simulink model "Component_1"  (R2024a)
settings: Solver=VariableStepAuto  StartTime=0.0  StopTime=10.0  RelTol=1e-3
undefined symbols (not defined in the file or in its folder): canChannel
libraries: canmsglib x4, canlib x2
settings Model: DataDictionary=BMS_System_dict1.sldd  Creator=hirah  LastModifiedBy=hirah

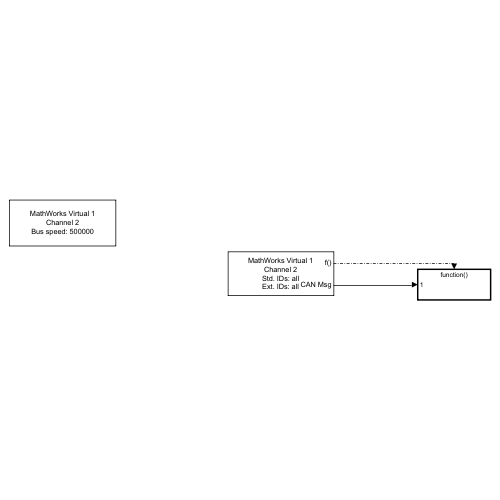
[thumbnail: Simulink's stored preview of the top-level diagram]
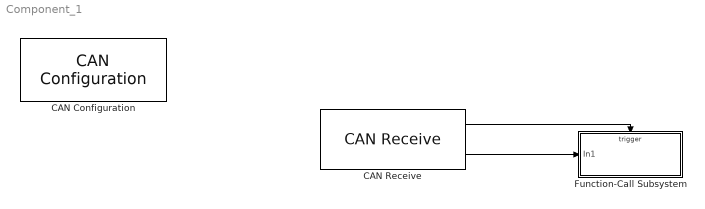
== system Component_1 ==
  CAN Configuration : canlib/CAN Configuration  BlockHandle=728.0002  Device=MathWorks Virtual 1 (Channel 2)  DeviceMenu=MathWorks Virtual 1 (Channel 2)  ObjConstructor=canChannel('MathWorks', 'Virtual 1', 2)  BusSpeed=500000  EnableBitParameters=off  AckMode=Normal
  CAN Receive : canlib/CAN Receive  BlockHandle=729.0002  Device=MathWorks Virtual 1 (Channel 2)  DeviceMenu=MathWorks Virtual 1 (Channel 2)  ObjConstructor=canChannel('MathWorks', 'Virtual 1', 2)  EnableStandardIDsFilter=off  StdIDsCombo=Allow all  StandardIDs=261  EnableExtendedIDsFilter=off  ExtIDsCombo=Allow all  ExtendedIDs=0  SampleTime=0.01  MsgsPerTimestep=all  InternalFilterUpdateStatus=on  BusOutput=off
  Function-Call Subsystem : Subsystem  TreatAsAtomicUnit=on
  wires:
  CAN Receive/1 -> Function-Call Subsystem/Trigger
  CAN Receive/2 -> Function-Call Subsystem/1(In1)

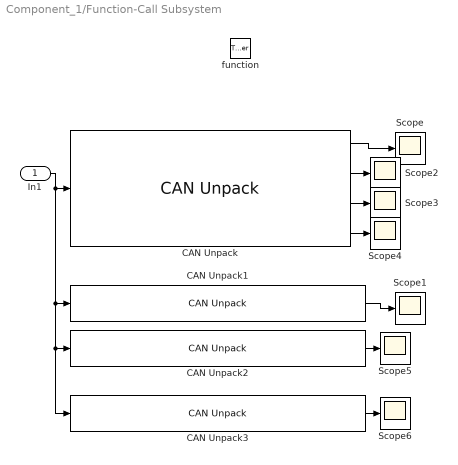
== system Component_1/Function-Call Subsystem ==
  In1 : Inport
  function : TriggerPort  TriggerType=function-call  VariantControl=(inherit)
  CAN Unpack : canmsglib/CAN Unpack  CANdbFile=C:\Users\hirah\Downloads\BMS_CAN_Database (5).dbc  MsgList=frmChargingControl  MsgName=frmChargingControl  MsgIDType=Standard (11-bit identifier)  MsgIdentifier=265  MsgLength=7  SignalInfo={ 'sigChargeModeRequest', '48', '8', 'LE', 'unsigned', 'Standard', '0', '1', '0', '0', '3'; 'sigChargeTerminationVoltage', '32', '16', 'LE', 'unsigned', 'Standard', '0', '0.1', '0', '0', '1000'; 'sigMaxChargeCurrent', '16', '16', 'LE', 'unsigned', 'Standard', '0', '0.1', '0', '0', '400'; 'sigMaxChargeVoltage', '0', '16', 'LE', 'unsigned', 'Standard', '0', '0.1', '0', '0', '1000' }  IDPort=off  TimestampPort=off  ErrorPort=off  RemotePort=off  LengthPort=off  StatusPort=off  ApplyMinMax=off
      settings: DataFormat=CANdb specified signals
  CAN Unpack1 : canmsglib/CAN Unpack  CANdbFile=C:\Users\hirah\Downloads\BMS_CAN_Database (5).dbc  MsgList=frmBMStoVCU  MsgName=frmBMStoVCU  MsgIDType=Standard (11-bit identifier)  MsgIdentifier=321  MsgLength=2  SignalInfo={ 'sigBMSOperatingMode', '0', '8', 'LE', 'unsigned', 'Standard', '0', '1', '0', '0', '5' }  IDPort=off  TimestampPort=off  ErrorPort=off  RemotePort=off  LengthPort=off  StatusPort=off  ApplyMinMax=off
  CAN Unpack2 : canmsglib/CAN Unpack  CANdbFile=C:\Users\hirah\Downloads\BMS_CAN_Database (5).dbc  MsgList=frmFaultStatus  MsgName=frmFaultStatus  MsgIDType=Standard (11-bit identifier)  MsgIdentifier=263  MsgLength=7  SignalInfo={ 'sigUndervoltageFault', '8', '8', 'LE', 'unsigned', 'Standard', '0', '1', '0', '0', '1' }  IDPort=off  TimestampPort=off  ErrorPort=off  RemotePort=off  LengthPort=off  StatusPort=off  ApplyMinMax=off
  CAN Unpack3 : canmsglib/CAN Unpack  CANdbFile=C:\Users\hirah\Downloads\BMS_CAN_Database (5).dbc  MsgList=frmSafetyBus  MsgName=frmSafetyBus  MsgIDType=Standard (11-bit identifier)  MsgIdentifier=261  MsgLength=4  SignalInfo={ 'sigChargeInhibit', '8', '8', 'LE', 'unsigned', 'Standard', '0', '1', '0', '0', '1' }  IDPort=off  TimestampPort=off  ErrorPort=off  RemotePort=off  LengthPort=off  StatusPort=off  ApplyMinMax=off
  Scope{,1..6} (7 alike) : Scope
  wires:
  In1/1 -> CAN Unpack3/1, CAN Unpack2/1, CAN Unpack1/1, CAN Unpack/1
  CAN Unpack/1 -> Scope/1
  CAN Unpack1/1 -> Scope1/1
  CAN Unpack/4 -> Scope4/1
  CAN Unpack/3 -> Scope3/1
  CAN Unpack/2 -> Scope2/1
  CAN Unpack2/1 -> Scope5/1
  CAN Unpack3/1 -> Scope6/1
